simulink model "sampleModel147_pp_difftest"  (R2021b)
settings: Solver=FixedStepAuto  StartTime=0.0  StopTime=10.0  RelTol=1e-3
libraries: simulink x2
settings Model: Creator=user  LastModifiedBy=cemery

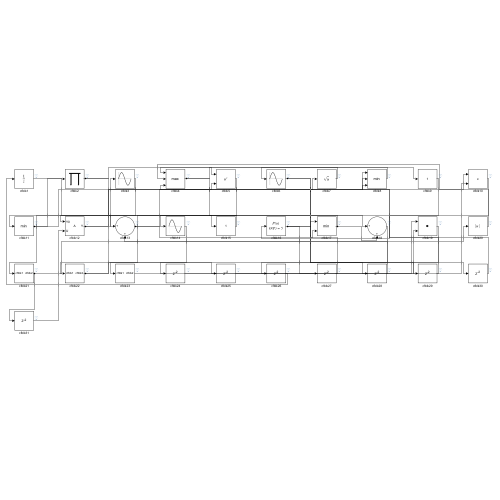
[thumbnail: Simulink's stored preview of the top-level diagram]
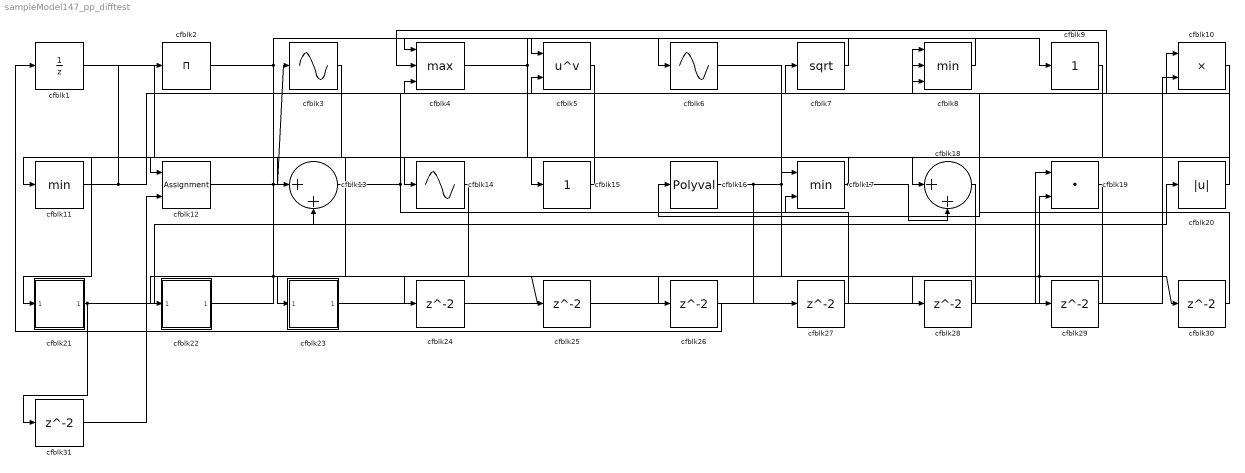
== system sampleModel147_pp_difftest ==
  cfblk1 : UnitDelay  HasFrameUpgradeWarning=on
  cfblk10 : Product
  cfblk11 : MinMax
  cfblk12 : Assignment  DiagnosticForDimensions=Warning  IndexOptions=Index vector (dialog)  Indices=1  OutputSizes=1
  cfblk13 : Sum  Inputs=|++
  cfblk14 : Sin  TimeSource=Use external signal  SampleTime=0
  cfblk15 : simulink/Math Operations/Slider Gain  gain=1  low=0  high=2
  cfblk16 : Polyval  Coefs=[ +2.081618890e-019, -1.441693666e-014, +4.719686976e-010, -8.536869453e-006, +1.621573104e-001, -8.087801117e+001 ]
  cfblk17 : MinMax  Inputs=2
  cfblk18 : Sum  Inputs=|++
  cfblk19 : DotProduct  InputSameDT=on  OutDataTypeStr=Inherit: Inherit via internal rule
  cfblk2 : Product  Inputs=*
  cfblk20 : Abs
  cfblk21 : Subsystem
  cfblk22 : Subsystem
  cfblk23 : Subsystem
  cfblk{24..31} (8 alike) : Delay  SampleTime=1
  cfblk3 : Sin  TimeSource=Use external signal  SampleTime=0
  cfblk4 : MinMax  Function=max  Inputs=3
  cfblk5 : Math  Operator=pow  SaturateOnIntegerOverflow=on
  cfblk6 : Sin  TimeSource=Use external signal  SampleTime=0
  cfblk7 : Sqrt  SaturateOnIntegerOverflow=on
  cfblk8 : MinMax  Inputs=3
  cfblk9 : simulink/Math Operations/Slider Gain  gain=1  low=0  high=2
  wires:
  cfblk9/1 -> cfblk16/1
  cfblk15/1 -> cfblk12/1
  cfblk7/1 -> cfblk4/1
  cfblk21/1(cfblk2) -> cfblk20/1, cfblk31/1
  cfblk12/1 -> cfblk3/1, cfblk8/1
  cfblk22/1(cfblk2) -> cfblk7/1, cfblk25/1
  cfblk23/1(cfblk2) -> cfblk19/2
  cfblk1/1 -> cfblk13/1
  cfblk20/1 -> cfblk4/2
  cfblk17/1 -> cfblk11/1, cfblk18/2
  cfblk19/1 -> cfblk22/1(cfblk1)
  cfblk16/1 -> cfblk8/2, cfblk28/1, cfblk27/1
  cfblk10/1 -> cfblk14/1
  cfblk2/1 -> cfblk5/1, cfblk15/1
  cfblk6/1 -> cfblk29/1, cfblk30/1
  cfblk5/1 -> cfblk23/1(cfblk1)
  cfblk3/1 -> cfblk21/1(cfblk1)
  cfblk11/1 -> cfblk5/2, cfblk2/1
  cfblk4/1 -> cfblk18/1, cfblk9/1
  cfblk8/1 -> cfblk6/1
  cfblk13/1 -> cfblk10/1, cfblk17/2
  cfblk14/1 -> cfblk24/1
  cfblk24/1 -> cfblk10/2
  cfblk25/1 -> cfblk19/1
  cfblk18/1 -> cfblk26/1
  cfblk26/1 -> cfblk1/1
  cfblk27/1 -> cfblk17/1
  cfblk28/1 -> cfblk13/2
  cfblk29/1 -> cfblk4/3
  cfblk30/1 -> cfblk8/3
  cfblk31/1 -> cfblk12/2

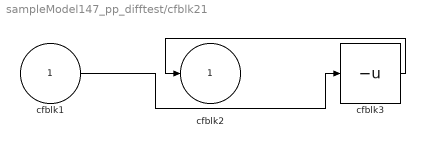
== system sampleModel147_pp_difftest/cfblk21 ==
  cfblk1 : Inport
  cfblk3 : UnaryMinus
  cfblk2 : Outport
  wires:
  cfblk3/1 -> cfblk2/1
  cfblk1/1 -> cfblk3/1

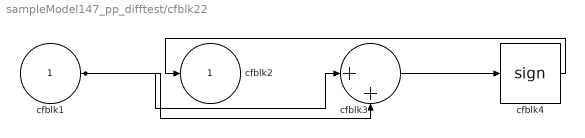
== system sampleModel147_pp_difftest/cfblk22 ==
  cfblk1 : Inport
  cfblk3 : Sum  Inputs=|++
  cfblk4 : Signum
  cfblk2 : Outport
  wires:
  cfblk4/1 -> cfblk2/1
  cfblk3/1 -> cfblk4/1
  cfblk1/1 -> cfblk3/1, cfblk3/2

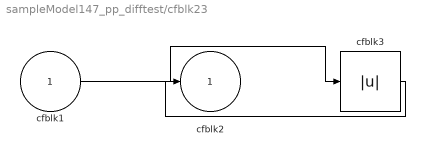
== system sampleModel147_pp_difftest/cfblk23 ==
  cfblk1 : Inport
  cfblk3 : Abs
  cfblk2 : Outport
  wires:
  cfblk1/1 -> cfblk3/1
  cfblk3/1 -> cfblk2/1
